simulink model "AS_SensorBank_VerifierModel"  (R2022b)
settings: Solver=VariableStepAuto  StartTime=0.0  StopTime=50  RelTol=1e-3
undefined symbols (not defined in the file): Blower_OutputDia, O2_OutputDia, PIDiameter
libraries: fl_lib x8, SimscapeFluids_lib x3, nesl_utility x2, simulink x1
settings Model: DataDictionary=AS_DataDictionary.sldd  Creator=CSN-Simulation  LastModifiedBy=MATLAB
settings DebuggingCC: UnconnectedInputMsg=warning  UnconnectedOutputMsg=warning  UnconnectedLineMsg=warning
settings ModelReferenceCC: EnableRefExpFcnMdlSchedulingChecks=on
settings RTWCC: DLArmComputeVersion=19.05

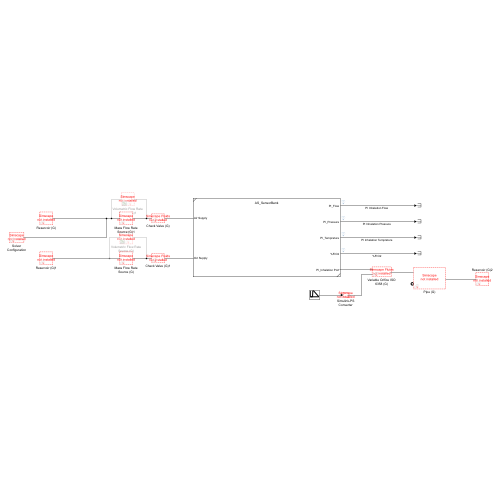
[thumbnail: Simulink's stored preview of the top-level diagram]
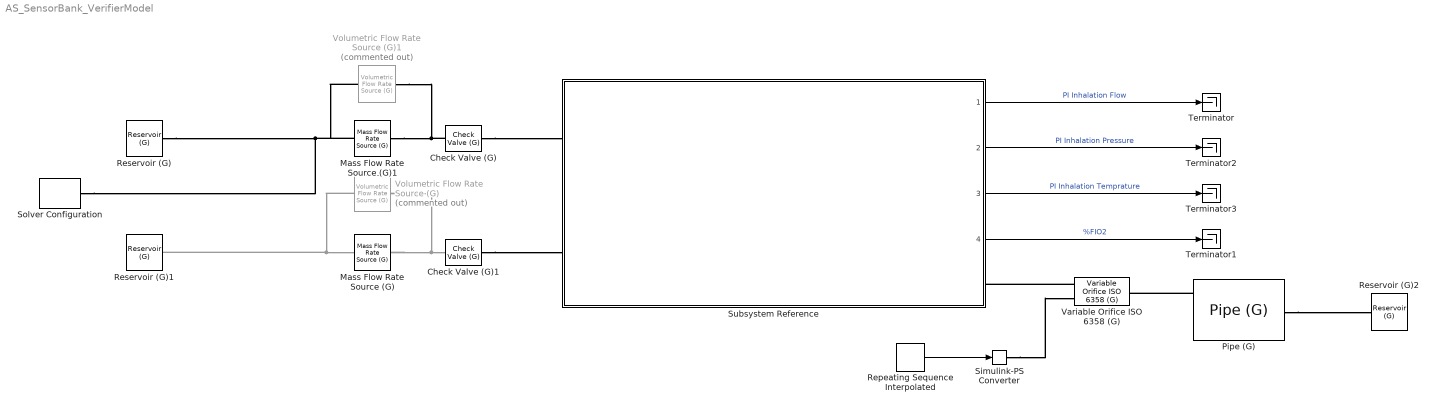
== system AS_SensorBank_VerifierModel ==
  Check Valve (G) : SimscapeFluids_lib/Gas/Valves & Orifices/Directional Control Valves/Check Valve (G)  pressure_spec=fluids.gas.enum.pressure_control_spec.dp  p_crack_differential=10 Pa  p_crack_gauge=0.1 MPa  press_max_differential=50 Pa  press_max_gauge=0.2 MPa  iso_cond_spec=fluids.gas.enum.iso_cond_spec.area  C_max=1.6 l/s/bar  C_min=1e-5 l/s/bar  B_crit=0.3  m=0.5  Cv_max=0.4  Cv_min=1e-6  Kv_max=0.3  Kv_min=1e-6  area_max=pi*(Blower_OutputDia/2)^2-pi*(2)^2 mm^2  area_leak=1 mm^2  area=pi*(Blower_OutputDia/2)^2 mm^2  smoothing_factor=0  B_lam=0.999  T0=293.15 K  rho0=1.185 kg/m^3
      settings: InternalSimscapePortConfiguration="{\"Bottom\":[],\"Left\":[{\"id\":\"A\",\"label\":\"A\",\"type\":\"foundation.gas.gas\"}],\"Right\":[{\"id\":\"B\",\"label\":\"B\",\"type\":\"foundation.gas.gas\"}],\"Top\":[]}"
  Check Valve (G)1 : SimscapeFluids_lib/Gas/Valves & Orifices/Directional Control Valves/Check Valve (G)  pressure_spec=fluids.gas.enum.pressure_control_spec.dp  p_crack_differential=10 Pa  p_crack_gauge=0.1 MPa  press_max_differential=50 Pa  press_max_gauge=0.2 MPa  iso_cond_spec=fluids.gas.enum.iso_cond_spec.area  C_max=pi*(O2_OutputDia/2)^2 l/s/bar  C_min=1e-5 l/s/bar  B_crit=0.3  m=0.5  Cv_max=0.4  Cv_min=1e-6  Kv_max=0.3  Kv_min=1e-6  area_max=pi*(O2_OutputDia/2)^2-pi*(2)^2 mm^2  area_leak=1e-12 mm^2  area=pi*(O2_OutputDia/2)^2 mm^2  smoothing_factor=0  B_lam=0.999  T0=293.15 K  rho0=1.185 kg/m^3
      settings: InternalSimscapePortConfiguration="{\"Bottom\":[],\"Left\":[{\"id\":\"A\",\"label\":\"A\",\"type\":\"foundation.gas.gas\"}],\"Right\":[{\"id\":\"B\",\"label\":\"B\",\"type\":\"foundation.gas.gas\"}],\"Top\":[]}"
  Mass Flow Rate Source (G) : fl_lib/Gas/Sources/Mass Flow Rate Source (G)  power_spec=foundation.enum.power_spec.isentropic  mass_flow=0.0002 kg/s  area_A=pi*(O2_OutputDia/2)^2 mm^2  area_B=pi*(O2_OutputDia/2)^2 mm^2
      settings: InternalSimscapePortConfiguration="{\"Bottom\":[],\"Left\":[{\"id\":\"A\",\"label\":\"A\",\"type\":\"foundation.gas.gas\"}],\"Right\":[{\"id\":\"B\",\"label\":\"B\",\"type\":\"foundation.gas.gas\"}],\"Top\":[]}"
  Mass Flow Rate Source (G)1 : fl_lib/Gas/Sources/Mass Flow Rate Source (G)  power_spec=foundation.enum.power_spec.isentropic  mass_flow=0.002 kg/s  area_A=pi*(Blower_OutputDia/2)^2 mm^2  area_B=pi*(Blower_OutputDia/2)^2 mm^2
      settings: InternalSimscapePortConfiguration="{\"Bottom\":[],\"Left\":[{\"id\":\"A\",\"label\":\"A\",\"type\":\"foundation.gas.gas\"}],\"Right\":[{\"id\":\"B\",\"label\":\"B\",\"type\":\"foundation.gas.gas\"}],\"Top\":[]}"
  Pipe (G) : fl_lib/Gas/Elements/Pipe (G)  length=4 m  area=pi*(PIDiameter/2)^2 mm^2  Dh=PIDiameter mm  length_add=0.1 m  roughness=15e-6 m  Re_lam=2000  Re_tur=4000  shape_factor=64  Nu_lam=3.66  p_I_specify=off  p_I_priority=High  p_I=0.101325 MPa  p_I_nominal_specify=off  p_I_nominal_unit=MPa  p_I_nominal_value=1  T_I_specify=off  T_I_priority=High  T_I=293.15 K  T_I_nominal_specify=off  T_I_nominal_unit=K  T_I_nominal_value=1  rho_pipe_specify=off  rho_pipe_priority=None  rho_pipe=1.2 kg/m^3  rho_pipe_nominal_specify=off  rho_pipe_nominal_unit=kg/m^3  rho_pipe_nominal_value=1
  Repeating Sequence Interpolated : simulink/Sources/Repeating Sequence Interpolated  OutValues=[0 0 1 1 0].'  TimeValues=[0 10 12 15 40 ].'  LookUpMeth=Interpolation-Use End Values  tsamp=0.1  OutMin=[]  OutMax=[]  OutDataTypeStr=double  OutputDataTypeScalingMode=double  OutDataType=fixdt(0,8)  OutScaling=2^-10
  Reservoir (G) : fl_lib/Gas/Elements/Reservoir (G)  pressure_spec=foundation.enum.pressure_spec.atmospheric  reservoir_pressure=0.101325 MPa  reservoir_temperature=T_room degC  area_A=pi*(Blower_OutputDia/2)^2 mm^2
  Reservoir (G)1 : fl_lib/Gas/Elements/Reservoir (G)  pressure_spec=foundation.enum.pressure_spec.atmospheric  reservoir_pressure=0.101325 MPa  reservoir_temperature=T_room degC  area_A=pi*(O2_OutputDia/2)^2 mm^2
  Reservoir (G)2 : fl_lib/Gas/Elements/Reservoir (G)  pressure_spec=foundation.enum.pressure_spec.atmospheric  reservoir_pressure=0.101325 MPa  reservoir_temperature=T_room degC  area_A=pi*(PIDiameter/2)^2 mm^2
  Simulink-PS Converter : nesl_utility/Simulink-PS Converter  PhysicalDomain=network_engine_domain  SubClassName=ps_input  LeftPortType=input  RightPortType=output  PseudoPeriodic=off  Frequencies=[]  NoiseDistribution=none  NoiseParameters=[]  Unit=1  AffineConversion=off  FilteringAndDerivatives=provide  SimscapeFilterOrder=1  InputFilterTimeConstant=0.001  UdotUserProvided=0
  Solver Configuration : nesl_utility/Solver Configuration  PhysicalDomain=network_engine_domain  SubClassName=solver  LeftPortType=input  RightPortType=generic  Tones=[]  Harmonics=[]  SimulateNoise=off  Profile=off  UseLocalSampling=off  EnableSwitchedLinearOptims=on  FrequencyDomain=off  UseCCode=off  RelTol=0.001  AbsTol=1e-06  MinStep=1e-09  ToWorkspace=off  RevertToSquareIcSolve=off  NumHomotopyIterations=100  PhasorMode=off  PhasorModeNumHarmonics=1  DoDC=on  ResidualTolerance=1e-09  UseLocalSolver=off  LocalSolverChoice=NE_BACKWARD_EULER_ADVANCER  LocalSolverSampleTime=0.001  DoFixedCost=off  MaxNonlinIter=3  MaxModeIter=2  ComputeImpulses=off  ImpulseIterations=2  LinearAlgebra=auto  EquationFormulation=NE_TIME_EF  DelaysMemoryBudget=1024  AutomaticFiltering=on  FilteringTimeConstant=0.001  PartitionStorageMethod=AS_NEEDED  PartitionMemoryBudget=1024  PartitionMethod=ROBUST
  Subsystem Reference : Subsystem  ReferencedSubsystem=AS_SensorBank
  Terminator{,1..3} (4 alike) : Terminator
  Variable Orifice ISO 6358 (G) : SimscapeFluids_lib/Gas/Valves & Orifices/Variable Orifice ISO 6358 (G)  iso_cond_spec=fluids.gas.enum.iso_cond_spec.area  iso_opening_spec_C=fluids.gas.enum.iso_opening_spec.linear  C_max=1.6 l/s/bar  C_min=1e-5 l/s/bar  B_crit=0.3  opening_C_TLU=0 : 0.2 : 1  C_TLU=[1e-05, .32, .64, .96, 1.28, 1.6] l/s/bar  B_crit_TLU=0.3 * ones(1, 6)  m=0.5  iso_opening_spec_Cv=fluids.gas.enum.iso_opening_spec.linear  Cv_max=0.4  Cv_min=1e-6  opening_Cv_TLU=0 : 0.2 : 1  Cv_TLU=[1e-06, .08, .16, .24, .32, .4]  iso_opening_spec_Kv=fluids.gas.enum.iso_opening_spec.linear  Kv_max=0.3  Kv_min=1e-6  opening_Kv_TLU=0 : 0.2 : 1  Kv_TLU=[1e-06, .06, .12, .18, .24, .3]  iso_opening_spec_area=fluids.gas.enum.iso_opening_spec.linear  restriction_area_max=pi*(PIDiameter/2)^2-pi*(2)^2 mm^2  restriction_area_min=1 mm^2  opening_area_TLU=0 : 0.2 : 1  restriction_area_TLU=[1e-10, 2e-06, 4e-06, 6e-06, 8e-06, 1e-05] m^2  area=pi*(PIDiameter/2)^2 mm^2  B_lam=0.999  T0=T_room degC  rho0=1.185 kg/m^3  smoothing_factor=0
      settings: InternalSimscapePortConfiguration="{\"Bottom\":[],\"Left\":[{\"id\":\"A\",\"label\":\"A\",\"type\":\"foundation.gas.gas\"},{\"id\":\"L\",\"label\":\"L\",\"type\":\"input\"}],\"Right\":[{\"id\":\"B\",\"label\":\"B\",\"type\":\"foundation.gas.gas\"}],\"Top\":[]}"
  Volumetric Flow Rate Source (G) : fl_lib/Gas/Sources/Volumetric Flow Rate Source (G)  Commented=on  power_spec=foundation.enum.power_spec.isentropic  volumetric_flow=80 lpm  area_A=pi*(O2_OutputDia/2)^2 mm^2  area_B=pi*(O2_OutputDia/2)^2 mm^2
      settings: InternalSimscapePortConfiguration="{\"Bottom\":[],\"Left\":[{\"id\":\"A\",\"label\":\"A\",\"type\":\"foundation.gas.gas\"}],\"Right\":[{\"id\":\"B\",\"label\":\"B\",\"type\":\"foundation.gas.gas\"}],\"Top\":[]}"
  Volumetric Flow Rate Source (G)1 : fl_lib/Gas/Sources/Volumetric Flow Rate Source (G)  Commented=on  power_spec=foundation.enum.power_spec.isentropic  volumetric_flow=160 lpm  area_A=pi*(Blower_OutputDia/2)^2 mm^2  area_B=pi*(Blower_OutputDia/2)^2 mm^2
      settings: InternalSimscapePortConfiguration="{\"Bottom\":[],\"Left\":[{\"id\":\"A\",\"label\":\"A\",\"type\":\"foundation.gas.gas\"}],\"Right\":[{\"id\":\"B\",\"label\":\"B\",\"type\":\"foundation.gas.gas\"}],\"Top\":[]}"
  wires:
  Subsystem Reference/1 -> Terminator/1  "PI Inhalation Flow"
  Subsystem Reference/2 -> Terminator2/1  "PI Inhalation Pressure"
  Subsystem Reference/3 -> Terminator3/1  "PI Inhalation Temprature"
  Subsystem Reference/4 -> Terminator1/1  "%FIO2"
  Repeating Sequence Interpolated/1 -> Simulink-PS Converter/1
  connections:
  Check Valve (G)/RConn1 -- Subsystem Reference/LConn1
  Check Valve (G)1/RConn1 -- Subsystem Reference/LConn2
  Check Valve (G)/LConn1 -- Volumetric Flow Rate Source (G)1/RConn1 -- Mass Flow Rate Source (G)1/RConn1
  Reservoir (G)/LConn1 -- Volumetric Flow Rate Source (G)1/LConn1 -- Mass Flow Rate Source (G)1/LConn1 -- Solver Configuration/RConn1
  Variable Orifice ISO 6358 (G)/LConn1 -- Subsystem Reference/RConn1
  Simulink-PS Converter/RConn1 -- Variable Orifice ISO 6358 (G)/LConn2
  Volumetric Flow Rate Source (G)/LConn1 -- Reservoir (G)1/LConn1 -- Mass Flow Rate Source (G)/LConn1
  Volumetric Flow Rate Source (G)/RConn1 -- Mass Flow Rate Source (G)/RConn1 -- Check Valve (G)1/LConn1
  Pipe (G)/LConn1 -- Variable Orifice ISO 6358 (G)/RConn1
  Pipe (G)/RConn1 -- Reservoir (G)2/LConn1
